simulink model "calibrate_gyro_24"  (R2024a)
settings: Solver=ode1  StartTime=0.0  StopTime=inf  FixedStep=0.01  RelTol=1e-3
model workspace (MAT data in the model file):
  alpha_gain = 0
undefined symbols (not defined in the file or in its folder): DiscIntNeverNeededParam, pin_number, state
libraries: ros2lib x17, slpidlib x2, dspstat3 x1, sharedutil x1, dspfdesign x1
settings Model: Creator=dsai9  LastModifiedBy=dsai9
settings OptimizationCC: EnhancedBackFolding=on  PassReuseOutputArgsAs=Individual arguments  ZeroExternalMemoryAtStartup=off  ZeroInternalMemoryAtStartup=off  MaxStackSize=64  OptimizeBlockOrder=speed  DifferentSizesBufferReuse=on  OptimizationCustomize=off  EfficientTunableParamExpr=on
settings DebuggingCC: ParameterTunabilityLossMsg=error
settings SFSimCC: MATLABDynamicMemAlloc=off
settings RTWCC: Description=Embedded Coder  SystemTargetFile=ert.tlc  HardwareBoard=Robot Operating System 2 (ROS 2)  TLCOptions="-aInlineSetEventsForThisBaseRateFcn=TLC_FALSE -aSuppressMultiTaskScheduler=TLC_FALSE  -aRateBasedStepFcn=0"  TemplateMakefile=ert_default_tmf  Toolchain=Colcon Tools  TargetLang=C++
settings CodeAppCC: ForceParamTrailComments=on  IgnoreCustomStorageClasses=off  OperatorAnnotations=on  SimulinkDataObjDesc=on  SFDataObjDesc=on  InsertBlockDesc=on
settings ERTTargetCC: CodeInterfacePackaging=C++ class  RootIOFormat=Structure reference

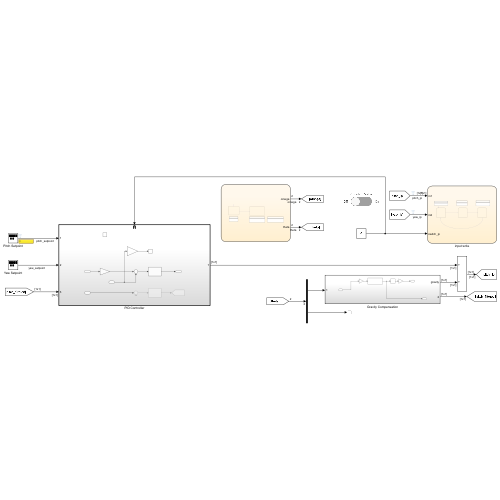
[thumbnail: Simulink's stored preview of the top-level diagram]
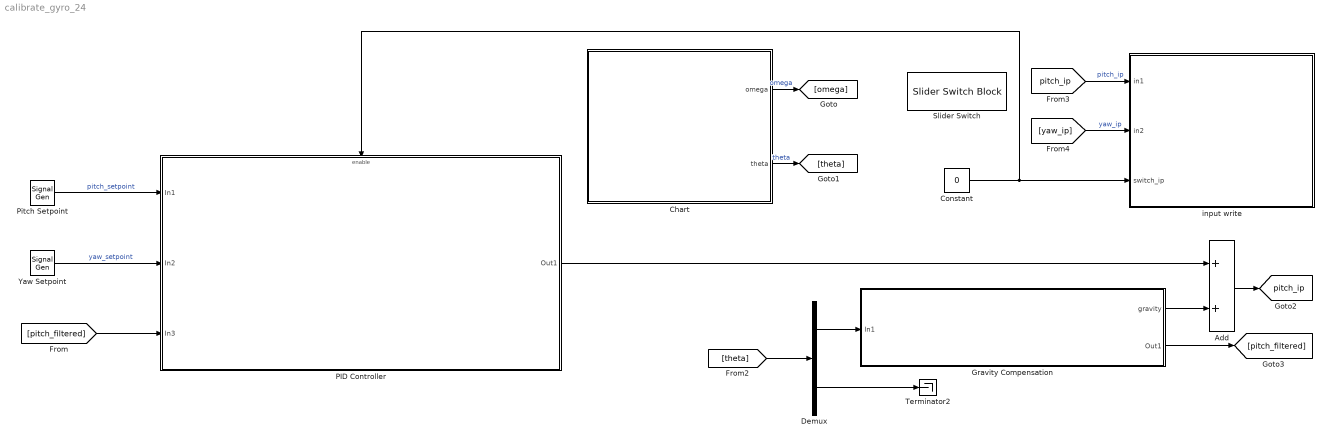
== system calibrate_gyro_24 ==
  Add : Sum
  Chart : Stateflow chart  TreatAsAtomicUnit=on
  Constant : Constant  Value=0
  Demux : Demux  Outputs=2
  Gravity Compensation : Subsystem
  PID Controller : Subsystem
  Pitch Setpoint : SignalGenerator  Amplitude=10  Frequency=0.01
  Slider Switch : SliderSwitchBlock
      settings: Values={{'Off', 'On'}, [0 1]}
  Terminator2 : Terminator
  Yaw Setpoint : SignalGenerator  Units=rad/sec
  input write : Stateflow chart  TreatAsAtomicUnit=on
  tag scope: pitch_ip=global
  wires:
  Chart/1(omega) -> [omega]  "omega"
  Chart/2(theta) -> [theta]  "theta"
  [pitch_ip] -> input write/1(in1)  "pitch_ip"
  [yaw_ip] -> input write/2(in2)  "yaw_ip"
  Constant/1 -> input write/3(switch_ip), PID Controller/Enable
  Yaw Setpoint/1 -> PID Controller/2(In2)  "yaw_setpoint"
  Pitch Setpoint/1 -> PID Controller/1(In1)  "pitch_setpoint"
  [pitch_filtered] -> PID Controller/3(In3)
  Add/1 -> [pitch_ip]
  [theta] -> Demux/1
  Demux/2 -> Terminator2/1
  PID Controller/1(Out1) -> Add/1
  Demux/1 -> Gravity Compensation/1(In1)
  Gravity Compensation/1(gravity) -> Add/2
  Gravity Compensation/2(Out1) -> [pitch_filtered]

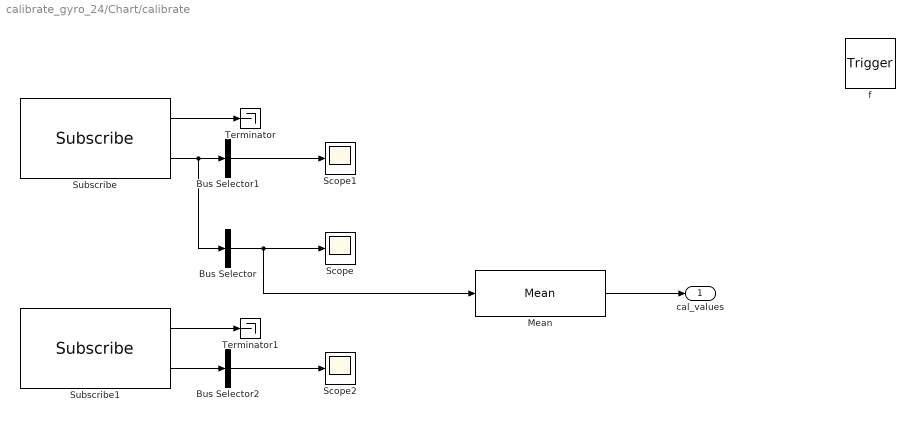
== system calibrate_gyro_24/Chart/calibrate ==
  f : TriggerPort  TriggerType=function-call  VariantControl=(inherit)
      settings: CopyFcn=Stateflow.SLINSF.SimulinkMan.removeBlockPreDeleteFcn  PreDeleteFcn=Stateflow.SLINSF.SimulinkMan.unsafePredeleteFcn
  Bus Selector : BusSelector  OutputSignals=angular_velocity.x,angular_velocity.y,angular_velocity.z  OutputAsBus=on
  Bus Selector1 : BusSelector  OutputSignals=linear_acceleration.x,linear_acceleration.y,linear_acceleration.z  OutputAsBus=on
  Bus Selector2 : BusSelector  OutputSignals=magnetic_field.x,magnetic_field.y,magnetic_field.z  OutputAsBus=on
  Mean : dspstat3/Mean  run=on  reset_popup=None  directionMode=Entire input  dimension=1  roiEnable=off  roiType=Rectangles  roiPortion=Entire ROI  roiOutput=Individual statistics for each ROI  roiFlag=off  roundingMode=Floor  overflowMode=off  outputDataTypeStr=Inherit: Same as accumulator  outputMin=[]  outputMax=[]  outputLastDataTypeStr=Inherit: Same as accumulator
  Scope : Scope
  Scope1 : Scope
  Scope2 : Scope
  Subscribe : ros2lib/Subscribe  topicSource=Select from ROS network  topic=/imu/data  messageType=sensor_msgs/Imu  sampleTime=-1  QOSHistory=Keep last  QOSDepth=1  QOSReliability=Reliable  QOSDurability=Volatile  QOSDeadline=Inf  QOSLifespan=Inf  QOSLiveliness=Automatic  QOSLeaseDuration=Inf  QOSAvoidROSNamespaceConventions=off
  Subscribe1 : ros2lib/Subscribe  topicSource=Select from ROS network  topic=/mag/data  messageType=sensor_msgs/MagneticField  sampleTime=-1  QOSHistory=Keep last  QOSDepth=1  QOSReliability=Reliable  QOSDurability=Volatile  QOSDeadline=Inf  QOSLifespan=Inf  QOSLiveliness=Automatic  QOSLeaseDuration=Inf  QOSAvoidROSNamespaceConventions=off
  Terminator : Terminator
  Terminator1 : Terminator
  cal_values : Outport  PortDimensions=3
  wires:
  Subscribe1/2 -> Bus Selector2/1
  Bus Selector2/1 -> Scope2/1
  Subscribe/1 -> Terminator/1
  Mean/1 -> cal_values/1
  Subscribe/2 -> Bus Selector/1, Bus Selector1/1
  Subscribe1/1 -> Terminator1/1
  Bus Selector/1 -> Mean/1, Scope/1
  Bus Selector1/1 -> Scope1/1

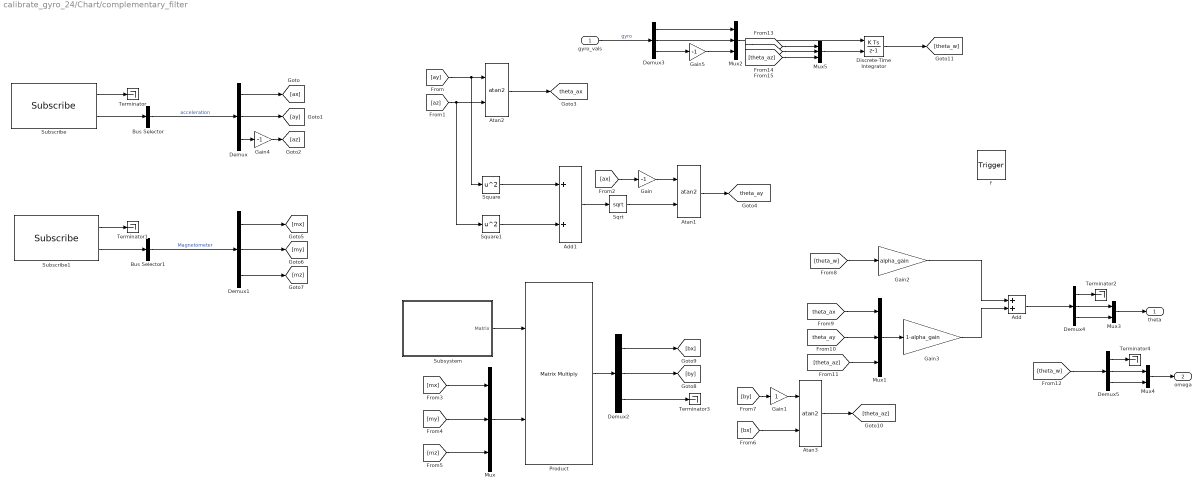
== system calibrate_gyro_24/Chart/complementary_filter ==
  gyro_vals : Inport  OutDataTypeStr=double  PortDimensions=3
  f : TriggerPort  TriggerType=function-call  VariantControl=(inherit)
      settings: CopyFcn=Stateflow.SLINSF.SimulinkMan.removeBlockPreDeleteFcn  PreDeleteFcn=Stateflow.SLINSF.SimulinkMan.unsafePredeleteFcn
  Add : Sum
  Add1 : Sum
  Atan1 : Trigonometry  Operator=atan2
  Atan2 : Trigonometry  Operator=atan2
  Atan3 : Trigonometry  Operator=atan2
  Bus Selector : BusSelector  OutputSignals=linear_acceleration.x,linear_acceleration.y,linear_acceleration.z  OutputAsBus=on
  Bus Selector1 : BusSelector  OutputSignals=magnetic_field.x,magnetic_field.y,magnetic_field.z  OutputAsBus=on
  Demux{,1..5} (6 alike) : Demux  Outputs=3
  Discrete-Time Integrator : DiscreteIntegrator  InitialConditionSource=external  SampleTime=-1  ICPrevOutput=DiscIntNeverNeededParam  ICPrevScaledInput=DiscIntNeverNeededParam
  Gain : Gain  Gain=-1
  Gain1 : Gain
  Gain2 : Gain  Gain=alpha_gain
  Gain3 : Gain  Gain=1-alpha_gain
  Gain4 : Gain  Gain=-1
  Gain5 : Gain  Gain=-1
  Mux{,1..2,5} (4 alike) : Mux  Inputs=3
  Mux3 : Mux  Inputs=2
  Mux4 : Mux  Inputs=2
  Product : Product  Multiplication=Matrix(*)
  Sqrt : Sqrt
  Square : Math  Operator=square
  Square1 : Math  Operator=square
  Subscribe : ros2lib/Subscribe  topicSource=Select from ROS network  topic=/imu/data  messageType=sensor_msgs/Imu  sampleTime=-1  QOSHistory=Keep last  QOSDepth=1  QOSReliability=Reliable  QOSDurability=Volatile  QOSDeadline=Inf  QOSLifespan=Inf  QOSLiveliness=Automatic  QOSLeaseDuration=Inf  QOSAvoidROSNamespaceConventions=off
  Subscribe1 : ros2lib/Subscribe  topicSource=Select from ROS network  topic=/mag/data  messageType=sensor_msgs/MagneticField  sampleTime=-1  QOSHistory=Keep last  QOSDepth=1  QOSReliability=Reliable  QOSDurability=Volatile  QOSDeadline=Inf  QOSLifespan=Inf  QOSLiveliness=Automatic  QOSLeaseDuration=Inf  QOSAvoidROSNamespaceConventions=off
  Subsystem : Subsystem
  Terminator{,1..4} (5 alike) : Terminator
  theta : Outport  PortDimensions=2
  omega : Outport  Port=2  PortDimensions=2
  tag scope: theta_ax=global, theta_ay=global
  wires:
  Subscribe/2 -> Bus Selector/1
  Subscribe1/2 -> Bus Selector1/1
  Bus Selector/1 -> Demux/1  "acceleration"
  Bus Selector1/1 -> Demux1/1  "Magnetometer"
  Subscribe/1 -> Terminator/1
  Subscribe1/1 -> Terminator1/1
  Demux/1 -> [ax]
  Demux/2 -> [ay]
  Demux/3 -> Gain4/1
  [ay] -> Square/1, Atan2/1
  [az] -> Square1/1, Atan2/2
  Atan2/1 -> [theta_ax]
  Square/1 -> Add1/1
  Square1/1 -> Add1/2
  Add1/1 -> Sqrt/1
  Sqrt/1 -> Atan1/2
  [ax] -> Gain/1
  Gain/1 -> Atan1/1
  Atan1/1 -> [theta_ay]
  Demux1/1 -> [mx]
  Demux1/2 -> [my]
  Demux1/3 -> [mz]
  Subsystem/1(Matrix) -> Product/1
  [mx] -> Mux/1
  [my] -> Mux/2
  [mz] -> Mux/3
  Mux/1 -> Product/2
  Product/1 -> Demux2/1
  Demux2/2 -> [by]
  Demux2/1 -> [bx]
  Demux2/3 -> Terminator3/1
  Gain1/1 -> Atan3/1
  [by] -> Gain1/1
  [bx] -> Atan3/2
  Atan3/1 -> [theta_az]
  Discrete-Time Integrator/1 -> [theta_w]
  [theta_w] -> Gain2/1
  [theta_ay] -> Mux1/2
  [theta_ax] -> Mux1/1
  [theta_az] -> Mux1/3
  Mux1/1 -> Gain3/1
  Gain2/1 -> Add/1
  Gain3/1 -> Add/2
  Gain4/1 -> [az]
  gyro_vals/1 -> Demux3/1  "gyro"
  Demux3/3 -> Gain5/1
  Gain5/1 -> Mux2/3
  Demux3/2 -> Mux2/2
  Demux3/1 -> Mux2/1
  Mux2/1 -> Discrete-Time Integrator/1
  Add/1 -> Demux4/1
  Mux3/1 -> theta/1
  Demux4/2 -> Mux3/1
  Demux4/3 -> Mux3/2
  Demux4/1 -> Terminator2/1
  Demux5/1 -> Terminator4/1
  Demux5/3 -> Mux4/2
  Demux5/2 -> Mux4/1
  [theta_w] -> Demux5/1
  Mux4/1 -> omega/1
  [theta_ax] -> Mux5/1
  [theta_ay] -> Mux5/2
  [theta_az] -> Mux5/3
  Mux5/1 -> Discrete-Time Integrator/2

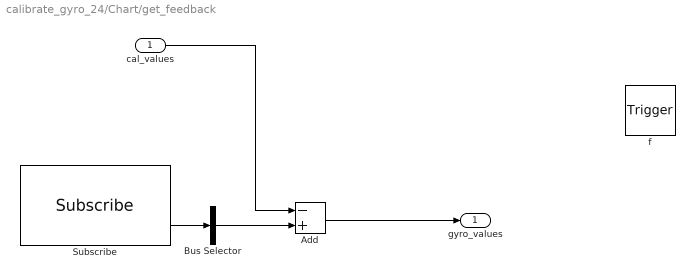
== system calibrate_gyro_24/Chart/get_feedback ==
  cal_values : Inport  OutDataTypeStr=double  PortDimensions=3
  f : TriggerPort  TriggerType=function-call  VariantControl=(inherit)
      settings: CopyFcn=Stateflow.SLINSF.SimulinkMan.removeBlockPreDeleteFcn  PreDeleteFcn=Stateflow.SLINSF.SimulinkMan.unsafePredeleteFcn
  Add : Sum  Inputs=-+
  Bus Selector : BusSelector  OutputSignals=angular_velocity.x,angular_velocity.y,angular_velocity.z  OutputAsBus=on
  Subscribe : ros2lib/Subscribe  topicSource=Select from ROS network  topic=/imu/data  messageType=sensor_msgs/Imu  sampleTime=-1  QOSHistory=Keep last  QOSDepth=1  QOSReliability=Reliable  QOSDurability=Volatile  QOSDeadline=Inf  QOSLifespan=Inf  QOSLiveliness=Automatic  QOSLeaseDuration=Inf  QOSAvoidROSNamespaceConventions=off
  gyro_values : Outport
  wires:
  Subscribe/2 -> Bus Selector/1
  Bus Selector/1 -> Add/2
  cal_values/1 -> Add/1
  Add/1 -> gyro_values/1

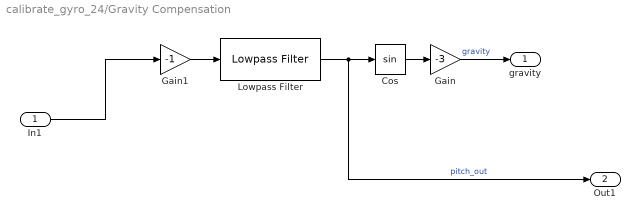
== system calibrate_gyro_24/Gravity Compensation ==
  In1 : Inport
  Cos : Trigonometry
  Gain : Gain  Gain=-3
  Gain1 : Gain  Gain=-1
  Lowpass Filter : dspfdesign/Lowpass Filter  FilterType=IIR  DesignForMinimumOrder=on  FilterOrder=1  PassbandFrequency=0.05  StopbandFrequency=0.06  PassbandRipple=1  StopbandAttenuation=80  SampleRateMode=Use normalized frequency (0 to 1)  SampleRate=100  SimulateUsing=Interpreted execution  roundingMode=Floor  coeffsDataTypeStr=fixdt(1,16)
  gravity : Outport
  Out1 : Outport  Port=2
  wires:
  In1/1 -> Gain1/1
  Cos/1 -> Gain/1
  Gain1/1 -> Lowpass Filter/1
  Gain/1 -> gravity/1  "gravity"
  Lowpass Filter/1 -> Out1/1, Cos/1  "pitch_out"

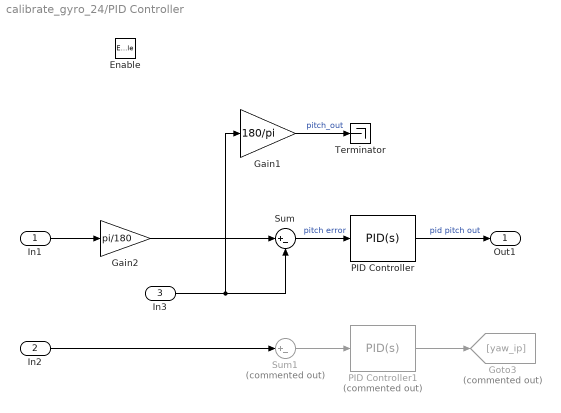
== system calibrate_gyro_24/PID Controller ==
  In1 : Inport
  In2 : Inport  Port=2
  In3 : Inport  Port=3
  Enable : EnablePort
  Gain1 : Gain  Gain=180/pi
  Gain2 : Gain  Gain=pi/180
  Goto3 : Goto  Commented=on  GotoTag=yaw_ip
  PID Controller : slpidlib/PID Controller  Controller=PID  Form=Parallel  TimeDomain=Continuous-time  UseExternalTs=off  SampleTime=-1  IntegratorMethod=Forward Euler  FilterMethod=Forward Euler  ControllerParametersSource=internal  P=20  I=6  UseKiTs=off  D=3  UseExternalDerivativeSource=off  N=100  UseFilter=on  TunerSelectOption=Transfer Function Based (PID Tuner App)  InitialConditionSource=internal  InitialConditionForIntegrator=0  InitialConditionForFilter=0  DifferentiatorICPrevScaledInput=0  ExternalReset=none  TrackingMode=off  Kt=1  LimitOutput=off  SatLimitsSource=internal  UpperSaturationLimit=inf  LowerSaturationLimit=-inf  LinearizeAsGain=on  AntiWindupMode=none  Kb=1  LimitIntegrator=off  UpperIntegratorSaturationLimit=inf  LowerIntegratorSaturationLimit=-inf  POutMin=[]  POutMax=[]  IOutMin=[]  IOutMax=[]  DOutMin=[]  DOutMax=[]  NOutMin=[]  NOutMax=[]  SumOutMin=[]  SumOutMax=[]  SaturationOutMin=[]  SaturationOutMax=[]  PParamMin=[]  PParamMax=[]  IParamMin=[]  IParamMax=[]  DParamMin=[]  DParamMax=[]  NParamMin=[]  NParamMax=[]  KbParamMin=[]  KbParamMax=[]  KtParamMin=[]  KtParamMax=[]  KbOutMin=[]  KbOutMax=[]  KtOutMin=[]  KtOutMax=[]  IntegratorOutMin=[]  IntegratorOutMax=[]  FilterOutMin=[]  FilterOutMax=[]  SumI1OutMin=[]  SumI1OutMax=[]  SumI2OutMin=[]  SumI2OutMax=[]  SumI3OutMin=[]  SumI3OutMax=[]  SumI4OutMin=[]  SumI4OutMax=[]  SumDOutMin=[]  SumDOutMax=[]  DifferentiatorOutMin=[]  DifferentiatorOutMax=[]  FilterDiffOutCoefMin=[]  FilterDiffOutCoefMax=[]  ReciprocalOutMin=[]  ReciprocalOutMax=[]  SumDenOutMin=[]  SumDenOutMax=[]  SumNumOutMin=[]  SumNumOutMax=[]  DivideOutMin=[]  DivideOutMax=[]  UdiffTsProdOutMin=[]  UdiffTsProdOutMax=[]  NTsProdOutMin=[]  NTsProdOutMax=[]  UintegralTsProdOutMin=[]  UintegralTsProdOutMax=[]  UngainTsProdOutMin=[]  UngainTsProdOutMax=[]  ClampingZeroOutDataTypeStr=Inherit: Inherit via back propagation  ClampingZeroOutMin=[]  ClampingZeroOutMax=[]  FilterDenConstantOutDataTypeStr=Inherit: Inherit via back propagation  FilterDenConstantOutMin=[]  FilterDenConstantOutMax=[]  PCopyOutDataTypeStr=Inherit: Inherit via back propagation  PCopyOutMin=[]  PCopyOutMax=[]  NCopyOutDataTypeStr=Inherit: Inherit via back propagation  NCopyOutMin=[]  NCopyOutMax=[]  IntegratorContinuousStateAttributes=''  IntegratorStateMustResolveToSignalObject=off  IntegratorRTWStateStorageClass=Auto  FilterContinuousStateAttributes=''  FilterStateMustResolveToSignalObject=off  FilterRTWStateStorageClass=Auto  ParallelPVariant=InternalParameters  IdealPVariant=Disabled  IVariant=InternalParameters  DVariant=InternalParameters  IntegratorVariant=Continuous  SatVariant=Disabled  AWVariant=Passthrough  PCopyVariant=Disabled  TRVariant=Disabled  FdbkBlocksVariant=Forward  IdealPFdbkVariant=Disabled  SatFdbkVariant=Disabled  DerivativeFilterVariant=ContFilter  NVariant=InternalParameters  NCopyVariant=Disabled  FilterICVariant=InternalICsFilter  IntegratorICVariant=InternalICs  ExternalResetVariant=Disabled  TRSumVariant=Passthrough  SumFdbkVariant=Disabled  SumVariant=Sum_PID  TsampFilterVariant=InternalTs  TsampNgainVariant=Passthrough  TsampIntegralVariant=Disabled_SignalSpec  ExternalSaturationOutDataTypeStr=Inherit: Same as second input  DerivativeSourceVariant=ErrorSignal
  PID Controller1 : slpidlib/PID Controller  Commented=on  Controller=PID  Form=Parallel  TimeDomain=Continuous-time  UseExternalTs=off  SampleTime=-1  IntegratorMethod=Forward Euler  FilterMethod=Forward Euler  ControllerParametersSource=internal  P=10  I=1  UseKiTs=off  D=0  UseExternalDerivativeSource=off  N=100  UseFilter=on  TunerSelectOption=Transfer Function Based (PID Tuner App)  InitialConditionSource=internal  InitialConditionForIntegrator=0  InitialConditionForFilter=0  DifferentiatorICPrevScaledInput=0  ExternalReset=none  TrackingMode=off  Kt=1  LimitOutput=off  SatLimitsSource=internal  UpperSaturationLimit=inf  LowerSaturationLimit=-inf  LinearizeAsGain=on  AntiWindupMode=none  Kb=1  LimitIntegrator=off  UpperIntegratorSaturationLimit=inf  LowerIntegratorSaturationLimit=-inf  POutMin=[]  POutMax=[]  IOutMin=[]  IOutMax=[]  DOutMin=[]  DOutMax=[]  NOutMin=[]  NOutMax=[]  SumOutMin=[]  SumOutMax=[]  SaturationOutMin=[]  SaturationOutMax=[]  PParamMin=[]  PParamMax=[]  IParamMin=[]  IParamMax=[]  DParamMin=[]  DParamMax=[]  NParamMin=[]  NParamMax=[]  KbParamMin=[]  KbParamMax=[]  KtParamMin=[]  KtParamMax=[]  KbOutMin=[]  KbOutMax=[]  KtOutMin=[]  KtOutMax=[]  IntegratorOutMin=[]  IntegratorOutMax=[]  FilterOutMin=[]  FilterOutMax=[]  SumI1OutMin=[]  SumI1OutMax=[]  SumI2OutMin=[]  SumI2OutMax=[]  SumI3OutMin=[]  SumI3OutMax=[]  SumI4OutMin=[]  SumI4OutMax=[]  SumDOutMin=[]  SumDOutMax=[]  DifferentiatorOutMin=[]  DifferentiatorOutMax=[]  FilterDiffOutCoefMin=[]  FilterDiffOutCoefMax=[]  ReciprocalOutMin=[]  ReciprocalOutMax=[]  SumDenOutMin=[]  SumDenOutMax=[]  SumNumOutMin=[]  SumNumOutMax=[]  DivideOutMin=[]  DivideOutMax=[]  UdiffTsProdOutMin=[]  UdiffTsProdOutMax=[]  NTsProdOutMin=[]  NTsProdOutMax=[]  UintegralTsProdOutMin=[]  UintegralTsProdOutMax=[]  UngainTsProdOutMin=[]  UngainTsProdOutMax=[]  ClampingZeroOutDataTypeStr=Inherit: Inherit via back propagation  ClampingZeroOutMin=[]  ClampingZeroOutMax=[]  FilterDenConstantOutDataTypeStr=Inherit: Inherit via back propagation  FilterDenConstantOutMin=[]  FilterDenConstantOutMax=[]  PCopyOutDataTypeStr=Inherit: Inherit via back propagation  PCopyOutMin=[]  PCopyOutMax=[]  NCopyOutDataTypeStr=Inherit: Inherit via back propagation  NCopyOutMin=[]  NCopyOutMax=[]  IntegratorContinuousStateAttributes=''  IntegratorStateMustResolveToSignalObject=off  IntegratorRTWStateStorageClass=Auto  FilterContinuousStateAttributes=''  FilterStateMustResolveToSignalObject=off  FilterRTWStateStorageClass=Auto  ParallelPVariant=InternalParameters  IdealPVariant=Disabled  IVariant=InternalParameters  DVariant=InternalParameters  IntegratorVariant=Continuous  SatVariant=Disabled  AWVariant=Passthrough  PCopyVariant=Disabled  TRVariant=Disabled  FdbkBlocksVariant=Forward  IdealPFdbkVariant=Disabled  SatFdbkVariant=Disabled  DerivativeFilterVariant=ContFilter  NVariant=InternalParameters  NCopyVariant=Disabled  FilterICVariant=InternalICsFilter  IntegratorICVariant=InternalICs  ExternalResetVariant=Disabled  TRSumVariant=Passthrough  SumFdbkVariant=Disabled  SumVariant=Sum_PID  TsampFilterVariant=InternalTs  TsampNgainVariant=Passthrough  TsampIntegralVariant=Disabled_SignalSpec  ExternalSaturationOutDataTypeStr=Inherit: Same as second input  DerivativeSourceVariant=ErrorSignal
  Sum : Sum  Inputs=|+-
  Sum1 : Sum  Commented=on  Inputs=|+-
  Terminator : Terminator
  Out1 : Outport
  wires:
  Sum1/1 -> PID Controller1/1
  Sum/1 -> PID Controller/1  "pitch error"
  PID Controller1/1 -> Goto3/1
  PID Controller/1 -> Out1/1  "pid pitch out"
  In1/1 -> Gain2/1
  In2/1 -> Sum1/1
  Gain1/1 -> Terminator/1  "pitch_out"
  Gain2/1 -> Sum/1
  In3/1 -> Gain1/1, Sum/2

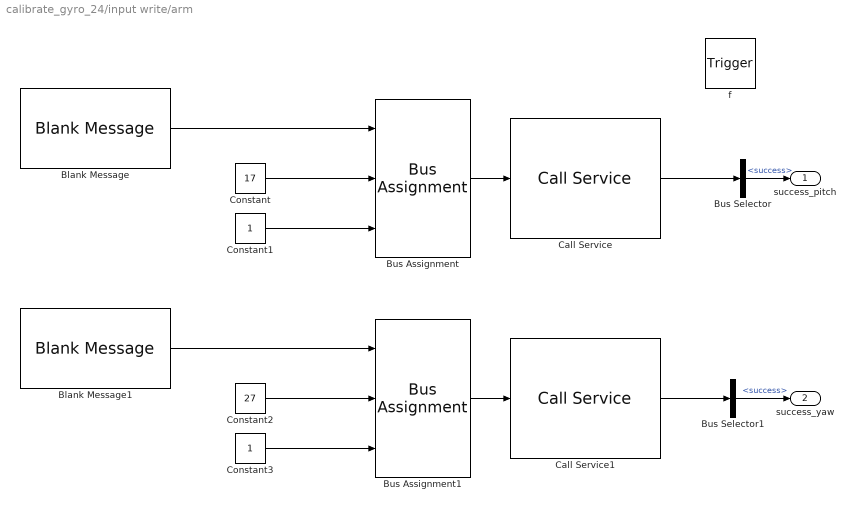
== system calibrate_gyro_24/input write/arm ==
  f : TriggerPort  TriggerType=function-call  VariantControl=(inherit)
      settings: CopyFcn=Stateflow.SLINSF.SimulinkMan.removeBlockPreDeleteFcn  PreDeleteFcn=Stateflow.SLINSF.SimulinkMan.unsafePredeleteFcn
  Blank Message : ros2lib/Blank Message  messageClass=Service Request  entityType=aerobot_interfaces/EscSrv  messageType=aerobot_interfaces/EscSrvRequest  SampleTime=inf
  Blank Message1 : ros2lib/Blank Message  messageClass=Service Request  entityType=aerobot_interfaces/EscSrv  messageType=aerobot_interfaces/EscSrvRequest  SampleTime=inf
  Bus Assignment : BusAssignment  AssignedSignals=pin_number,state
  Bus Assignment1 : BusAssignment  AssignedSignals=pin_number,state
  Bus Selector : BusSelector  OutputSignals=success
  Bus Selector1 : BusSelector  OutputSignals=success
  Call Service : ros2lib/Call Service  topicSource=Select from ROS network  service=/arm_pitch  serviceType=aerobot_interfaces/EscSrv  connectionTimeout=5  ShowErrorCodeOutput=off  legacyBusStruct=off  QOSHistory=Keep last  QOSDepth=1  QOSReliability=Reliable  QOSDurability=Volatile  QOSDeadline=Inf  QOSLifespan=Inf  QOSLiveliness=Automatic  QOSLeaseDuration=Inf  QOSAvoidROSNamespaceConventions=off
  Call Service1 : ros2lib/Call Service  topicSource=Select from ROS network  service=/arm_pitch  serviceType=aerobot_interfaces/EscSrv  connectionTimeout=5  ShowErrorCodeOutput=off  legacyBusStruct=off  QOSHistory=Keep last  QOSDepth=1  QOSReliability=Reliable  QOSDurability=Volatile  QOSDeadline=Inf  QOSLifespan=Inf  QOSLiveliness=Automatic  QOSLeaseDuration=Inf  QOSAvoidROSNamespaceConventions=off
  Constant : Constant  Value=17  OutDataTypeStr=int8
  Constant1 : Constant  OutDataTypeStr=boolean
  Constant2 : Constant  Value=27  OutDataTypeStr=int8
  Constant3 : Constant  OutDataTypeStr=boolean
  success_pitch : Outport
  success_yaw : Outport  Port=2
  wires:
  Blank Message/1 -> Bus Assignment/1
  Bus Assignment/1 -> Call Service/1
  Constant/1 -> Bus Assignment/2
  Constant1/1 -> Bus Assignment/3
  Constant3/1 -> Bus Assignment1/3
  Blank Message1/1 -> Bus Assignment1/1
  Bus Assignment1/1 -> Call Service1/1
  Constant2/1 -> Bus Assignment1/2
  Call Service/1 -> Bus Selector/1
  Bus Selector/1 -> success_pitch/1  "<success>"
  Call Service1/1 -> Bus Selector1/1
  Bus Selector1/1 -> success_yaw/1  "<success>"

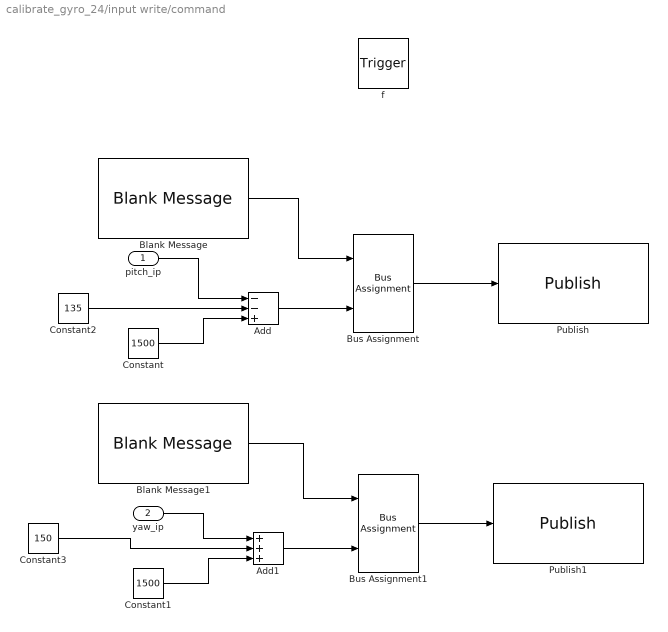
== system calibrate_gyro_24/input write/command ==
  pitch_ip : Inport  OutDataTypeStr=double  PortDimensions=1
  yaw_ip : Inport  Port=2  OutDataTypeStr=double  PortDimensions=1
  f : TriggerPort  TriggerType=function-call  VariantControl=(inherit)
      settings: CopyFcn=Stateflow.SLINSF.SimulinkMan.removeBlockPreDeleteFcn  PreDeleteFcn=Stateflow.SLINSF.SimulinkMan.unsafePredeleteFcn
  Add : Sum  Inputs=--+
  Add1 : Sum  Inputs=+++
  Blank Message : ros2lib/Blank Message  messageClass=Message  entityType=std_msgs/Float64  messageType=std_msgs/Float64  SampleTime=inf
  Blank Message1 : ros2lib/Blank Message  messageClass=Message  entityType=std_msgs/Float64  messageType=std_msgs/Float64  SampleTime=inf
  Bus Assignment : BusAssignment  AssignedSignals=data
  Bus Assignment1 : BusAssignment  AssignedSignals=data
  Constant : Constant  Value=1500
  Constant1 : Constant  Value=1500
  Constant2 : Constant  Value=135
  Constant3 : Constant  Value=150
  Publish : ros2lib/Publish  topicSource=Select from ROS network  topic=/esc_command1  messageType=std_msgs/Float64  QOSHistory=Keep last  QOSDepth=1  QOSReliability=Reliable  QOSDurability=Volatile  QOSDeadline=Inf  QOSLifespan=Inf  QOSLiveliness=Automatic  QOSLeaseDuration=Inf  QOSAvoidROSNamespaceConventions=off
  Publish1 : ros2lib/Publish  topicSource=Select from ROS network  topic=/esc_command2  messageType=std_msgs/Float64  QOSHistory=Keep last  QOSDepth=1  QOSReliability=Reliable  QOSDurability=Volatile  QOSDeadline=Inf  QOSLifespan=Inf  QOSLiveliness=Automatic  QOSLeaseDuration=Inf  QOSAvoidROSNamespaceConventions=off
  wires:
  Bus Assignment/1 -> Publish/1
  Blank Message/1 -> Bus Assignment/1
  Add/1 -> Bus Assignment/2
  Constant/1 -> Add/3
  pitch_ip/1 -> Add/1
  yaw_ip/1 -> Add1/1
  Constant1/1 -> Add1/3
  Add1/1 -> Bus Assignment1/2
  Blank Message1/1 -> Bus Assignment1/1
  Bus Assignment1/1 -> Publish1/1
  Constant2/1 -> Add/2
  Constant3/1 -> Add1/2

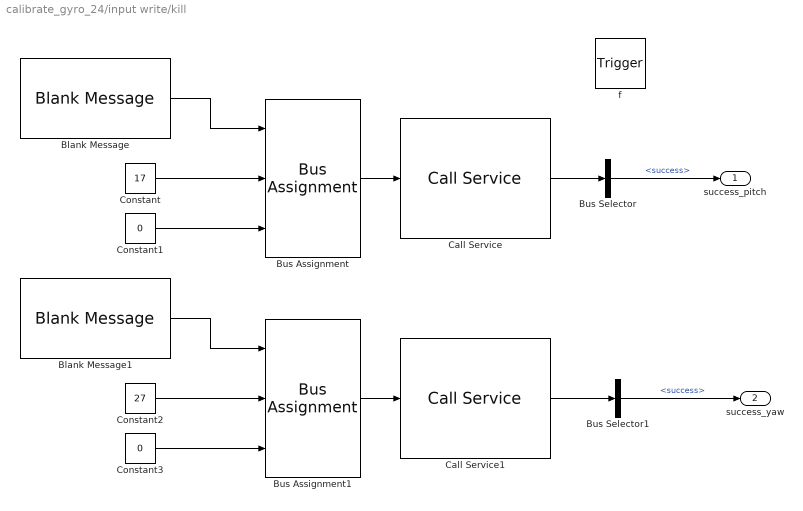
== system calibrate_gyro_24/input write/kill ==
  f : TriggerPort  TriggerType=function-call  VariantControl=(inherit)
      settings: CopyFcn=Stateflow.SLINSF.SimulinkMan.removeBlockPreDeleteFcn  PreDeleteFcn=Stateflow.SLINSF.SimulinkMan.unsafePredeleteFcn
  Blank Message : ros2lib/Blank Message  messageClass=Service Request  entityType=aerobot_interfaces/EscSrv  messageType=aerobot_interfaces/EscSrvRequest  SampleTime=inf
  Blank Message1 : ros2lib/Blank Message  messageClass=Service Request  entityType=aerobot_interfaces/EscSrv  messageType=aerobot_interfaces/EscSrvRequest  SampleTime=inf
  Bus Assignment : BusAssignment  AssignedSignals=pin_number,state
  Bus Assignment1 : BusAssignment  AssignedSignals=pin_number,state
  Bus Selector : BusSelector  OutputSignals=success
  Bus Selector1 : BusSelector  OutputSignals=success
  Call Service : ros2lib/Call Service  topicSource=Select from ROS network  service=/arm_pitch  serviceType=aerobot_interfaces/EscSrv  connectionTimeout=5  ShowErrorCodeOutput=off  legacyBusStruct=off  QOSHistory=Keep last  QOSDepth=1  QOSReliability=Reliable  QOSDurability=Volatile  QOSDeadline=Inf  QOSLifespan=Inf  QOSLiveliness=Automatic  QOSLeaseDuration=Inf  QOSAvoidROSNamespaceConventions=off
  Call Service1 : ros2lib/Call Service  topicSource=Select from ROS network  service=/arm_pitch  serviceType=aerobot_interfaces/EscSrv  connectionTimeout=5  ShowErrorCodeOutput=off  legacyBusStruct=off  QOSHistory=Keep last  QOSDepth=1  QOSReliability=Reliable  QOSDurability=Volatile  QOSDeadline=Inf  QOSLifespan=Inf  QOSLiveliness=Automatic  QOSLeaseDuration=Inf  QOSAvoidROSNamespaceConventions=off
  Constant : Constant  Value=17  OutDataTypeStr=int8
  Constant1 : Constant  Value=0  OutDataTypeStr=boolean
  Constant2 : Constant  Value=27  OutDataTypeStr=int8
  Constant3 : Constant  Value=0  OutDataTypeStr=boolean
  success_pitch : Outport
  success_yaw : Outport  Port=2
  wires:
  Blank Message/1 -> Bus Assignment/1
  Bus Assignment/1 -> Call Service/1
  Constant/1 -> Bus Assignment/2
  Constant1/1 -> Bus Assignment/3
  Call Service1/1 -> Bus Selector1/1
  Constant3/1 -> Bus Assignment1/3
  Blank Message1/1 -> Bus Assignment1/1
  Bus Assignment1/1 -> Call Service1/1
  Constant2/1 -> Bus Assignment1/2
  Call Service/1 -> Bus Selector/1
  Bus Selector/1 -> success_pitch/1  "<success>"
  Bus Selector1/1 -> success_yaw/1  "<success>"

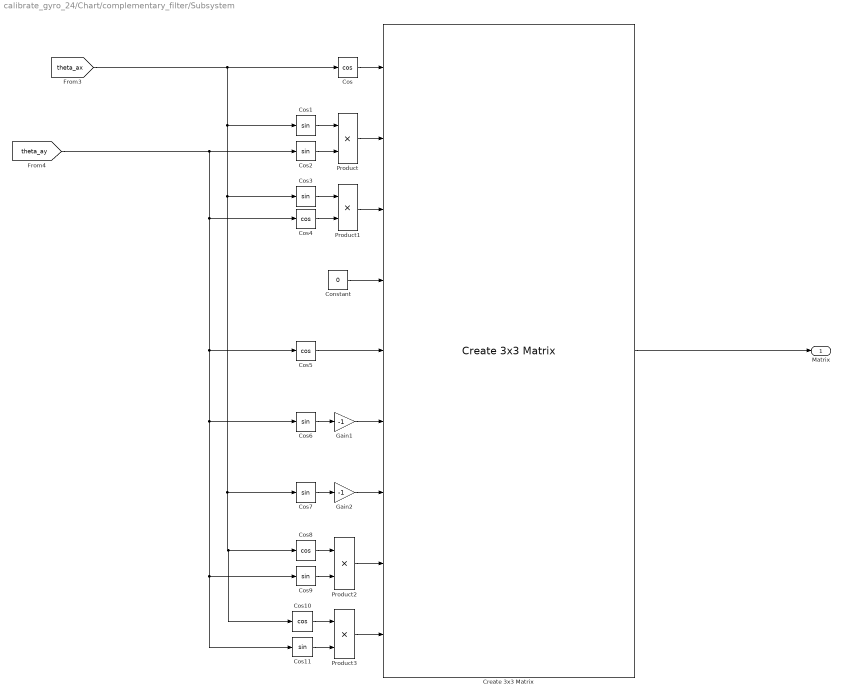
== system calibrate_gyro_24/Chart/complementary_filter/Subsystem ==
  Constant : Constant  Value=0
  Cos{,4..5,8,10} (5 alike) : Trigonometry  Operator=cos
  Cos{1..3,6..7,9,11} (7 alike) : Trigonometry
  Create 3x3 Matrix : sharedutil/Create 3x3 Matrix  aMode=aMode
      settings: LibrarySourceBlock=aerolibutil/Create 3x3 Matrix
  Gain1 : Gain  Gain=-1
  Gain2 : Gain  Gain=-1
  Product{,1..3} (4 alike) : Product
  Matrix : Outport  PortDimensions=[3,3]
  wires:
  Gain2/1 -> Create 3x3 Matrix/7
  Cos7/1 -> Gain2/1
  Cos8/1 -> Product2/1
  [theta_ax] -> Cos/1, Cos10/1, Cos8/1, Cos7/1, Cos3/1, Cos1/1
  Product3/1 -> Create 3x3 Matrix/9
  Cos11/1 -> Product3/2
  Cos9/1 -> Product2/2
  Cos10/1 -> Product3/1
  Constant/1 -> Create 3x3 Matrix/4
  Product/1 -> Create 3x3 Matrix/2
  Cos3/1 -> Product1/1
  [theta_ay] -> Cos5/1, Cos6/1, Cos11/1, Cos9/1, Cos4/1, Cos2/1
  Cos1/1 -> Product/1
  Cos6/1 -> Gain1/1
  Cos/1 -> Create 3x3 Matrix/1
  Product1/1 -> Create 3x3 Matrix/3
  Gain1/1 -> Create 3x3 Matrix/6
  Cos5/1 -> Create 3x3 Matrix/5
  Cos4/1 -> Product1/2
  Product2/1 -> Create 3x3 Matrix/8
  Cos2/1 -> Product/2
  Create 3x3 Matrix/1 -> Matrix/1

== stateflow chart calibrate_gyro_24/input write ==
  state [success_pitch,success_yaw] = kill [function]
  state command(pitch_ip,yaw_ip) [function]
  state [success_pitch,success_yaw] = arm [function]
  state arm_state
    entry:
    [ps, ys] = arm()
    move = 1
  state Command_state
    during:
    command(in1, in2)
  state kill_state
    entry:
    [ps, ys] = kill()
  (default) -> arm_state
  arm_state -> Command_state : [move == 1]
  Command_state -> kill_state : [switch_ip ==  0]
  kill_state -> arm_state : [switch_ip == 1]
  data: success_pitch function_output; success_yaw function_output; pitch_ip function_input double size=1; yaw_ip function_input double size=1; success_pitch function_output; success_yaw function_output; in1 input; in2 input; ys local; ps local; move local; switch_ip input

== stateflow chart calibrate_gyro_24/Chart ==
  state calibrate_start
    entry:
    calibrated = 0;
    i = 0;
    during:
    cal_values = calibrate();
    i = i + 1;
    if i == 100;
    disp('Calibration Done')
    calibrated = 1;
    end
  state orientation_calculation
    during:
    gyro_values = get_feedback(cal_values);
    [theta, omega] = complementary_filter(gyro_values);
  state cal_values = calibrate [function]
  state gyro_values = get_feedback(cal_values) [function]
  state [theta,omega] = complementary_filter(gyro_vals) [function]
  (default) -> calibrate_start
  calibrate_start -> orientation_calculation : [calibrated==1]
  data: cal_values function_output size=3; cal_values function_input double size=3; gyro_values function_output; gyro_vals function_input double size=3; theta function_output size=2; omega function_output size=2; calibrated local; i local; cal_values local; omega output; gyro_values local; theta output
